simulink library "guidanceLawPathFollowingController"  (R2020a)
settings: Solver=VariableStepAuto  StartTime=0.0  StopTime=10.0  RelTol=1e-3
libraries: pathFollowingController_cl x1, spoolingController_cl x1
settings Model: Creator=Ayaz  LastModifiedBy=Ayaz

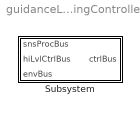
== system guidanceLawPathFollowingController ==
  Subsystem : Subsystem

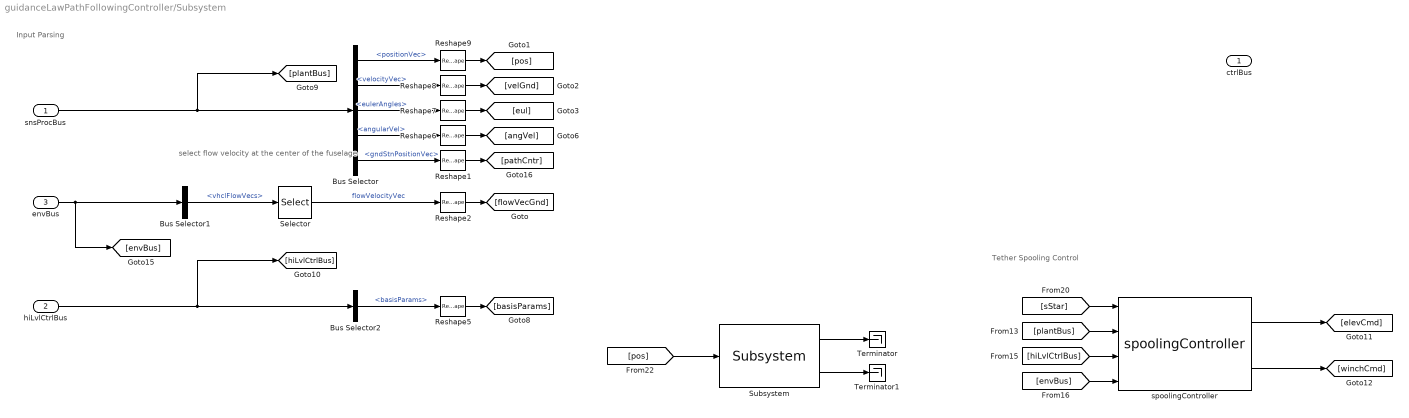
== system guidanceLawPathFollowingController/Subsystem ==
  note: select flow velocity at the center of the fuselage
  note: Tether Spooling Control
  note: Input Parsing
  snsProcBus : Inport  OutDataTypeStr=Bus: sensorsProcessingBus
  hiLvlCtrlBus : Inport  Port=2  OutDataTypeStr=Bus: hiLvlCtrlBus
  envBus : Inport  Port=3  OutDataTypeStr=Bus: envBus
  Bus Selector : BusSelector  OutputSignals=positionVec,velocityVec,eulerAngles,angularVel,gndStnPositionVec
  Bus Selector1 : BusSelector  OutputSignals=vhclFlowVecs
  Bus Selector2 : BusSelector  OutputSignals=basisParams
  Reshape{1..2,5..9} (7 alike) : Reshape  OutputDimensionality=Column vector (2-D)
  Selector : Selector  NumberOfDimensions=2  InputPortWidth=3  IndexOptions=Select all,Index vector (dialog)  Indices=[1 3],5  OutputSizes=1,1
  Subsystem : pathFollowingController_cl/pathFollowingController/Subsystem  SystemSampleTime=-1  Latency=0  AutoFrameSizeCalculation=off
  Terminator : Terminator
  Terminator1 : Terminator
  spoolingController : spoolingController_cl/spoolingController  SystemSampleTime=-1  Latency=0  AutoFrameSizeCalculation=off
  ctrlBus : Outport  OutDataTypeStr=Bus: fltCtrlBus  VectorParamsAs1DForOutWhenUnconnected=off
  wires:
  Bus Selector/1 -> Reshape9/1  "<positionVec>"
  Bus Selector/2 -> Reshape8/1  "<velocityVec>"
  hiLvlCtrlBus/1 -> Bus Selector2/1, [hiLvlCtrlBus]
  Reshape8/1 -> [velGnd]
  snsProcBus/1 -> Bus Selector/1, [plantBus]
  Bus Selector/4 -> Reshape6/1  "<angularVel>"
  Reshape9/1 -> [pos]
  Reshape6/1 -> [angVel]
  Bus Selector2/1 -> Reshape5/1  "<basisParams>"
  Reshape7/1 -> [eul]
  Selector/1 -> Reshape2/1  "flowVelocityVec"
  Bus Selector/3 -> Reshape7/1  "<eulerAngles>"
  Reshape5/1 -> [basisParams]
  Reshape1/1 -> [pathCntr]
  Bus Selector/5 -> Reshape1/1  "<gndStnPositionVec>"
  Bus Selector1/1 -> Selector/1  "<vhclFlowVecs>"
  envBus/1 -> [envBus], Bus Selector1/1
  Reshape2/1 -> [flowVecGnd]
  Subsystem/2 -> Terminator1/1
  Subsystem/1 -> Terminator/1
  [pos] -> Subsystem/1
  [plantBus] -> spoolingController/2
  spoolingController/1 -> [elevCmd]
  [sStar] -> spoolingController/1
  spoolingController/2 -> [winchCmd]
  [envBus] -> spoolingController/4
  [hiLvlCtrlBus] -> spoolingController/3
